simulink model "ask1"  (R2016a)
settings: Solver=VariableStepAuto  StartTime=0.0  StopTime=0.005  RelTol=1e-3
values from neighbouring files (symbols this model uses):
  k = 182    [ex1.m]
  kd = 1.946*10^(-3)    (= 0.001946)    [ex1.m]
  kp = 1    [ex1.m]
libraries: simulink x1
settings Model: Creator=JIM  LastModifiedBy=JIM

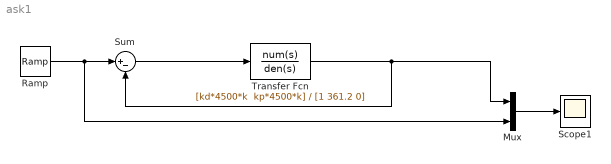
== system ask1 ==
  Mux : Mux  Inputs=2
  Ramp : simulink/Sources/Ramp  slope=1  start=0  X0=0
  Scope1 : Scope
  Sum : Sum  Inputs=|+-
  Transfer Fcn : TransferFcn  Numerator="[kd*4500*k  kp*4500*k]"  Denominator=[1 361.2 0]
  wires:
  Transfer Fcn/1 -> Sum/2, Mux/1
  Sum/1 -> Transfer Fcn/1
  Ramp/1 -> Mux/2, Sum/1
  Mux/1 -> Scope1/1
